simulink model "Reference_Speed_Generator"  (R2016b)
settings: Solver=FixedStepAuto  StartTime=0.0  StopTime=1500  FixedStep=0.001  RelTol=1e-3
PostLoadFcn:
  | addpath('./GUIFiles');
  | 
  | load default_gui_data.mat
  | 
  | %Load GUI
  | h_sync_gui = optiTruckGUI;
InitFcn:
  | % Call parameters initialization function
  | % run optiTruck_init_sim.m;
StopFcn:
  | %optiTruck_post_sim;
  | %optiTruck_plot_sim;
undefined symbols (not defined in the file or in its folder): DiscIntNeverNeededParam
settings Model: Creator=engin  LastModifiedBy=engin.ozatay
settings DataIOCC: SaveFormat=StructureWithTime  SaveOutput=off  SaveTime=off
settings OptimizationCC: BlockReduction=off  BufferReuse=off  LifeSpan=inf
settings DebuggingCC: AlgebraicLoopMsg=none  UnconnectedInputMsg=none  UnconnectedOutputMsg=none  UnconnectedLineMsg=none  SFExecutionAtInitializationDiag=none
settings HardwareCC: ProdBitPerSizeT=32  ProdBitPerPtrDiffT=32  ProdWordSize=32  ProdHWDeviceType=Specified

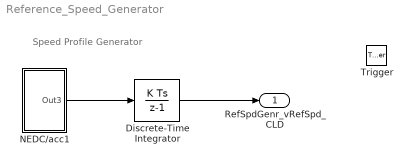
== system Reference_Speed_Generator ==
  note: Speed Profile Generator
  Trigger : TriggerPort  TriggerType=function-call  VariantControl=Variant  PortDimensions=1
  Discrete-Time Integrator : DiscreteIntegrator  SampleTime=-1  ICPrevOutput=DiscIntNeverNeededParam  ICPrevScaledInput=DiscIntNeverNeededParam
  NEDC/acc1 : Subsystem
  RefSpdGenr_vRefSpd_CLD : Outport
  wires:
  Discrete-Time Integrator/1 -> RefSpdGenr_vRefSpd_CLD/1
  NEDC/acc1/1(Out3) -> Discrete-Time Integrator/1

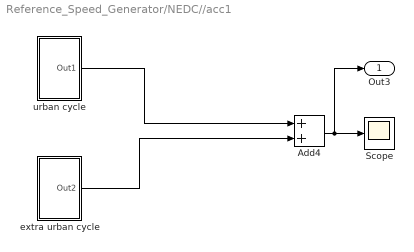
== system Reference_Speed_Generator/NEDC//acc1 ==
  Add4 : Sum
  Scope : Scope
  extra urban cycle : Subsystem
  urban cycle : Subsystem
  Out3 : Outport
  wires:
  urban cycle/1(Out1) -> Add4/1
  extra urban cycle/1(Out2) -> Add4/2
  Add4/1 -> Scope/1, Out3/1

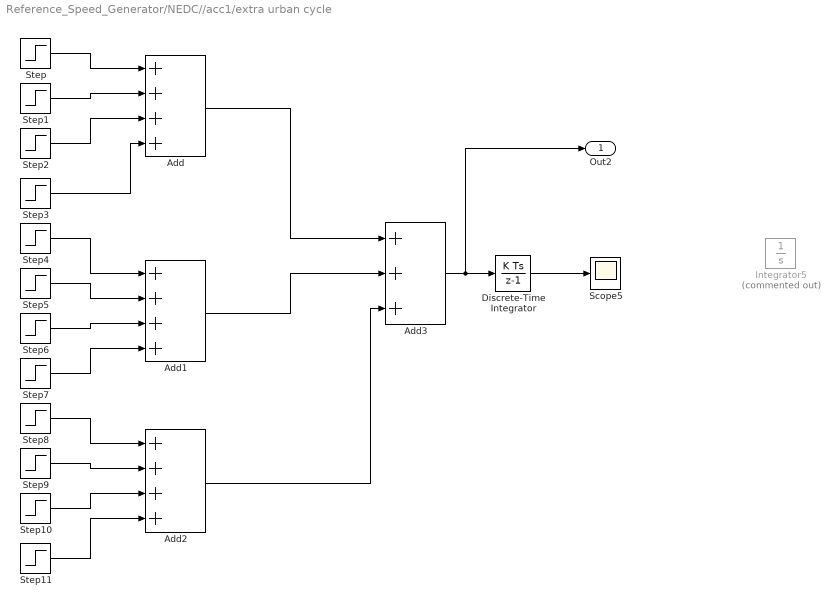
== system Reference_Speed_Generator/NEDC//acc1/extra urban cycle ==
  Add : Sum  Inputs=++++
  Add1 : Sum  Inputs=++++
  Add2 : Sum  Inputs=++++
  Add3 : Sum  Inputs=+++
  Discrete-Time Integrator : DiscreteIntegrator  SampleTime=-1  ICPrevOutput=DiscIntNeverNeededParam  ICPrevScaledInput=DiscIntNeverNeededParam
  Integrator5 : Integrator  Commented=on
  Scope5 : Scope
  Step : Step  Time=800  After=1.522/3.6  ZeroCross=off
  Step1 : Step  Time=846  After=-1.522/3.6  ZeroCross=off
  Step10 : Step  Time=1155  After=2.666/3.6  ZeroCross=off
  Step11 : Step  Time=900  After=2.5/3.6  ZeroCross=off
  Step2 : Step  Time=892  After=-2.5/3.6  ZeroCross=off
  Step3 : Step  Time=975  After=1.33/3.6  ZeroCross=off
  Step4 : Step  Time=990  After=-1.33/3.6  ZeroCross=off
  Step5 : Step  Time=1030  After=1/3.6  ZeroCross=off
  Step6 : Step  Time=1060  After=-1/3.6  ZeroCross=off
  Step7 : Step  Time=1090  After=2/3.6  ZeroCross=off
  Step8 : Step  Time=1100  After=-2/3.6  ZeroCross=off
  Step9 : Step  Time=1110  After=-2.666/3.6  ZeroCross=off
  Out2 : Outport
  wires:
  Step/1 -> Add/1
  Step1/1 -> Add/2
  Step2/1 -> Add/3
  Step3/1 -> Add/4
  Step4/1 -> Add1/1
  Step5/1 -> Add1/2
  Step6/1 -> Add1/3
  Step7/1 -> Add1/4
  Step8/1 -> Add2/1
  Step9/1 -> Add2/2
  Step10/1 -> Add2/3
  Add/1 -> Add3/1
  Add1/1 -> Add3/2
  Add2/1 -> Add3/3
  Discrete-Time Integrator/1 -> Scope5/1
  Add3/1 -> Discrete-Time Integrator/1, Out2/1
  Step11/1 -> Add2/4

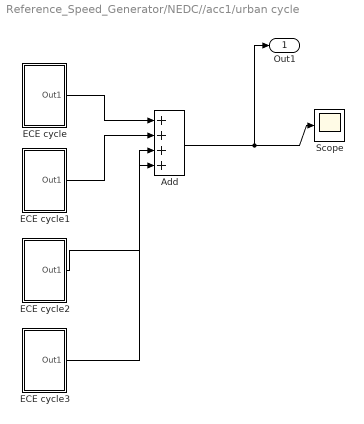
== system Reference_Speed_Generator/NEDC//acc1/urban cycle ==
  Add : Sum  Inputs=++++
  ECE cycle : Subsystem
  ECE cycle1 : Subsystem
  ECE cycle2 : Subsystem
  ECE cycle3 : Subsystem
  Scope : Scope
  Out1 : Outport
  wires:
  ECE cycle/1(Out1) -> Add/1
  ECE cycle1/1(Out1) -> Add/2
  Add/1 -> Scope/1, Out1/1
  ECE cycle2/1(Out1) -> Add/3
  ECE cycle3/1(Out1) -> Add/4

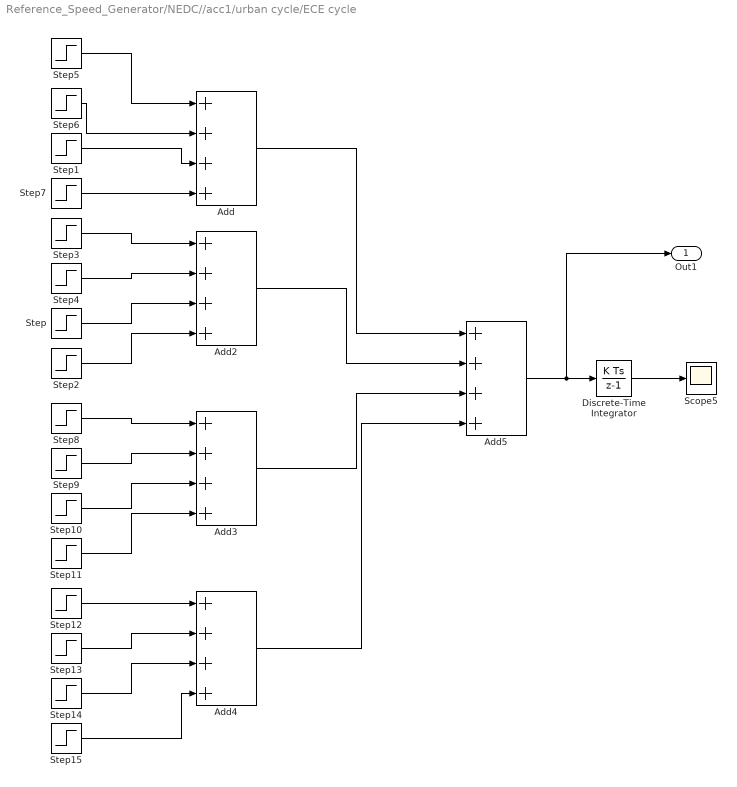
== system Reference_Speed_Generator/NEDC//acc1/urban cycle/ECE cycle ==
  Add{,2..5} (5 alike) : Sum  Inputs=++++
  Discrete-Time Integrator : DiscreteIntegrator  SampleTime=-1  ICPrevOutput=DiscIntNeverNeededParam  ICPrevScaledInput=DiscIntNeverNeededParam
  Scope5 : Scope
  Step : Step  Time=85  After=-3.2/3.6  ZeroCross=off
  Step1 : Step  Time=23  After=-3/3.6  ZeroCross=off
  Step10 : Step  Time=134  After=1.6/3.6  ZeroCross=off
  Step11 : Step  Time=144  After=-1.6/3.6  ZeroCross=off
  Step12 : Step  Time=155  After=-1.875/3.6  ZeroCross=off
  Step13 : Step  Time=163  After=1.875/3.6  ZeroCross=off
  Step14 : Step  Time=178  After=-3.5/3.6  ZeroCross=off
  Step15 : Step  Time=188  After=3.5/3.6  ZeroCross=off
  Step2 : Step  Time=95  After=3.2/3.6  ZeroCross=off
  Step3 : Step  Time=50  After=3.2/3.6  ZeroCross=off
  Step4 : Step  Time=60  After=-3.2/3.6  ZeroCross=off
  Step5 : Step  Time=10  After=3/3.6  ZeroCross=off
  Step6 : Step  Time=15  After=-3/3.6  ZeroCross=off
  Step7 : Step  Time=28  After=3/3.6  ZeroCross=off
  Step8 : Step  Time=117  After=2/3.6  ZeroCross=off
  Step9 : Step  Time=134  After=-2/3.6  ZeroCross=off
  Out1 : Outport
  wires:
  Step5/1 -> Add/1
  Step6/1 -> Add/2
  Step1/1 -> Add/3
  Step7/1 -> Add/4
  Step3/1 -> Add2/1
  Step4/1 -> Add2/2
  Step/1 -> Add2/3
  Step2/1 -> Add2/4
  Step8/1 -> Add3/1
  Step9/1 -> Add3/2
  Step10/1 -> Add3/3
  Step11/1 -> Add3/4
  Step12/1 -> Add4/1
  Step13/1 -> Add4/2
  Step14/1 -> Add4/3
  Step15/1 -> Add4/4
  Discrete-Time Integrator/1 -> Scope5/1
  Add5/1 -> Discrete-Time Integrator/1, Out1/1
  Add/1 -> Add5/1
  Add2/1 -> Add5/2
  Add3/1 -> Add5/3
  Add4/1 -> Add5/4

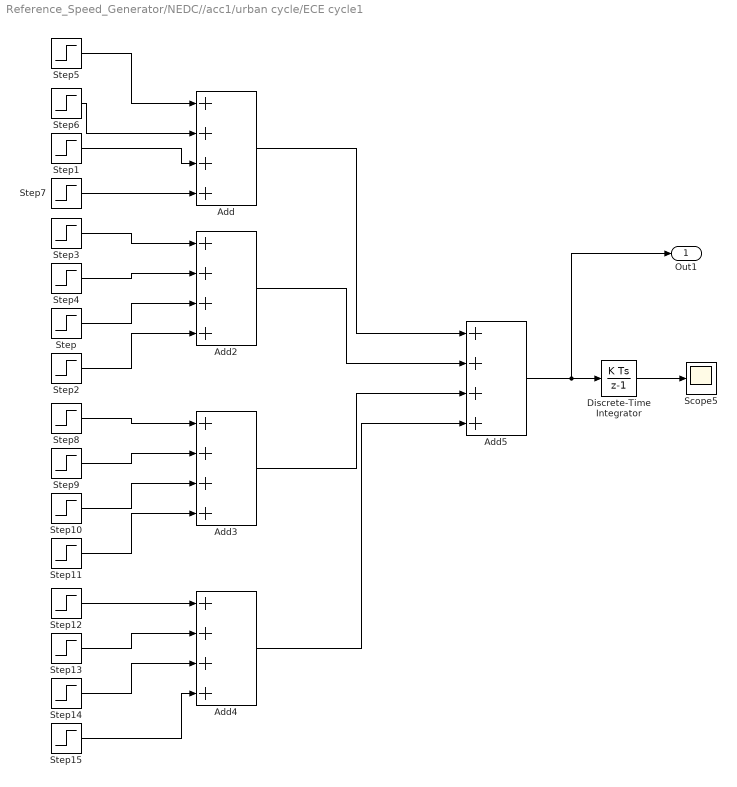
== system Reference_Speed_Generator/NEDC//acc1/urban cycle/ECE cycle1 ==
  Add{,2..5} (5 alike) : Sum  Inputs=++++
  Discrete-Time Integrator : DiscreteIntegrator  SampleTime=-1  ICPrevOutput=DiscIntNeverNeededParam  ICPrevScaledInput=DiscIntNeverNeededParam
  Scope5 : Scope
  Step : Step  Time=85+200  After=-3.2/3.6  ZeroCross=off
  Step1 : Step  Time=23+200  After=-3/3.6  ZeroCross=off
  Step10 : Step  Time=134+200  After=1.6/3.6  ZeroCross=off
  Step11 : Step  Time=144+200  After=-1.6/3.6  ZeroCross=off
  Step12 : Step  Time=155+200  After=-1.875/3.6  ZeroCross=off
  Step13 : Step  Time=163+200  After=1.875/3.6  ZeroCross=off
  Step14 : Step  Time=178+200  After=-3.5/3.6  ZeroCross=off
  Step15 : Step  Time=188+200  After=3.5/3.6  ZeroCross=off
  Step2 : Step  Time=95+200  After=3.2/3.6  ZeroCross=off
  Step3 : Step  Time=50+200  After=3.2/3.6  ZeroCross=off
  Step4 : Step  Time=60+200  After=-3.2/3.6  ZeroCross=off
  Step5 : Step  Time=10+200  After=3/3.6  ZeroCross=off
  Step6 : Step  Time=15+200  After=-3/3.6  ZeroCross=off
  Step7 : Step  Time=28+200  After=3/3.6  ZeroCross=off
  Step8 : Step  Time=117+200  After=2/3.6  ZeroCross=off
  Step9 : Step  Time=134+200  After=-2/3.6  ZeroCross=off
  Out1 : Outport
  wires:
  Step5/1 -> Add/1
  Step6/1 -> Add/2
  Step1/1 -> Add/3
  Step7/1 -> Add/4
  Step3/1 -> Add2/1
  Step4/1 -> Add2/2
  Step/1 -> Add2/3
  Step2/1 -> Add2/4
  Step8/1 -> Add3/1
  Step9/1 -> Add3/2
  Step10/1 -> Add3/3
  Step11/1 -> Add3/4
  Step12/1 -> Add4/1
  Step13/1 -> Add4/2
  Step14/1 -> Add4/3
  Step15/1 -> Add4/4
  Discrete-Time Integrator/1 -> Scope5/1
  Add5/1 -> Discrete-Time Integrator/1, Out1/1
  Add/1 -> Add5/1
  Add2/1 -> Add5/2
  Add3/1 -> Add5/3
  Add4/1 -> Add5/4

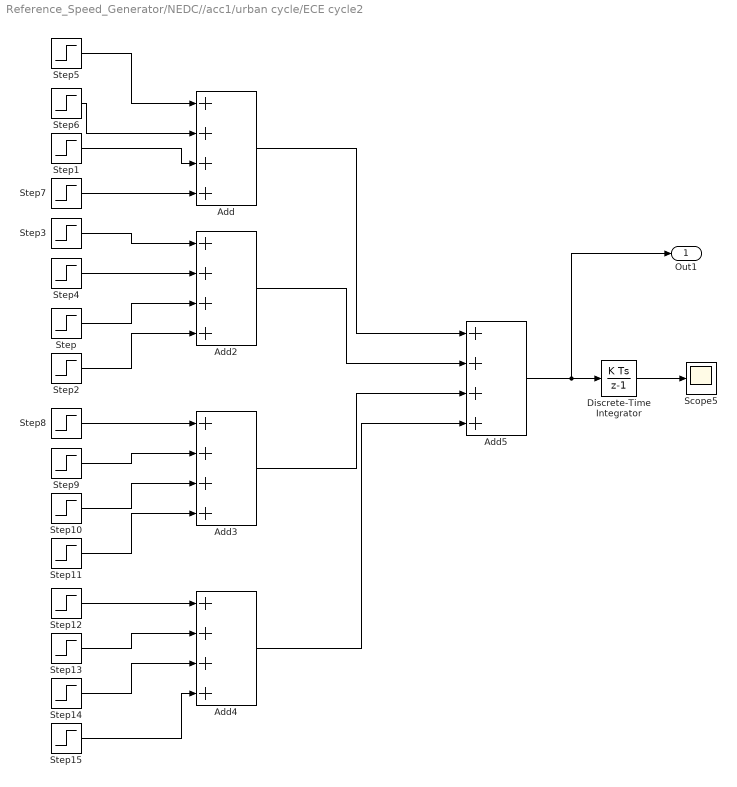
== system Reference_Speed_Generator/NEDC//acc1/urban cycle/ECE cycle2 ==
  Add{,2..5} (5 alike) : Sum  Inputs=++++
  Discrete-Time Integrator : DiscreteIntegrator  SampleTime=-1  ICPrevOutput=DiscIntNeverNeededParam  ICPrevScaledInput=DiscIntNeverNeededParam
  Scope5 : Scope
  Step : Step  Time=85+400  After=-3.2/3.6  ZeroCross=off
  Step1 : Step  Time=23+400  After=-3/3.6  ZeroCross=off
  Step10 : Step  Time=134+400  After=1.6/3.6  ZeroCross=off
  Step11 : Step  Time=144+400  After=-1.6/3.6  ZeroCross=off
  Step12 : Step  Time=155+400  After=-1.875/3.6  ZeroCross=off
  Step13 : Step  Time=163+400  After=1.875/3.6  ZeroCross=off
  Step14 : Step  Time=178+400  After=-3.5/3.6  ZeroCross=off
  Step15 : Step  Time=188+400  After=3.5/3.6  ZeroCross=off
  Step2 : Step  Time=95+400  After=3.2/3.6  ZeroCross=off
  Step3 : Step  Time=50+400  After=3.2/3.6  ZeroCross=off
  Step4 : Step  Time=60+400  After=-3.2/3.6  ZeroCross=off
  Step5 : Step  Time=10+400  After=3/3.6  ZeroCross=off
  Step6 : Step  Time=15+400  After=-3/3.6  ZeroCross=off
  Step7 : Step  Time=28+400  After=3/3.6  ZeroCross=off
  Step8 : Step  Time=117+400  After=2/3.6  ZeroCross=off
  Step9 : Step  Time=134+400  After=-2/3.6  ZeroCross=off
  Out1 : Outport
  wires:
  Step5/1 -> Add/1
  Step6/1 -> Add/2
  Step1/1 -> Add/3
  Step7/1 -> Add/4
  Step3/1 -> Add2/1
  Step4/1 -> Add2/2
  Step/1 -> Add2/3
  Step2/1 -> Add2/4
  Step8/1 -> Add3/1
  Step9/1 -> Add3/2
  Step10/1 -> Add3/3
  Step11/1 -> Add3/4
  Step12/1 -> Add4/1
  Step13/1 -> Add4/2
  Step14/1 -> Add4/3
  Step15/1 -> Add4/4
  Discrete-Time Integrator/1 -> Scope5/1
  Add5/1 -> Discrete-Time Integrator/1, Out1/1
  Add/1 -> Add5/1
  Add2/1 -> Add5/2
  Add3/1 -> Add5/3
  Add4/1 -> Add5/4

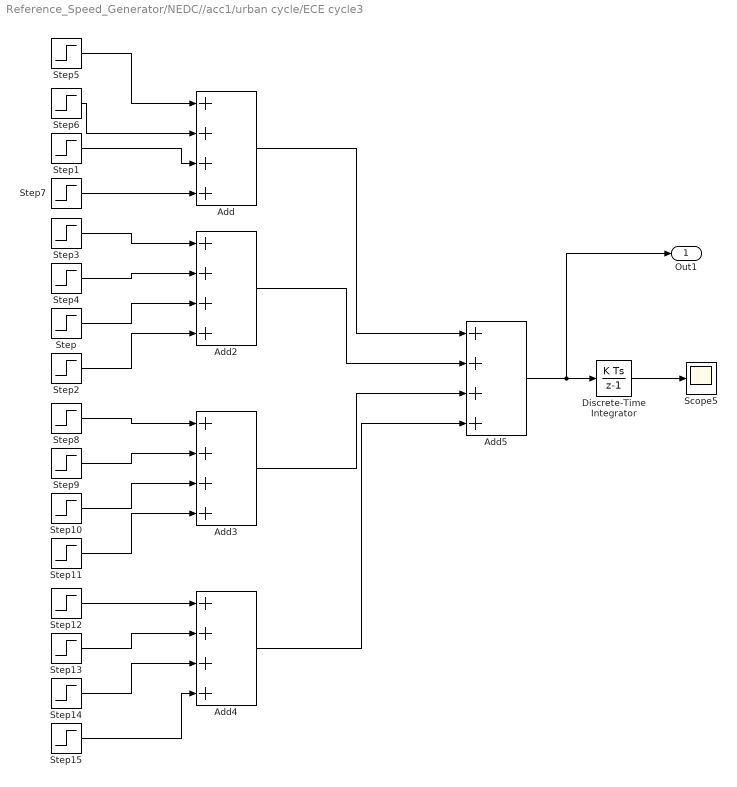
== system Reference_Speed_Generator/NEDC//acc1/urban cycle/ECE cycle3 ==
  Add{,2..5} (5 alike) : Sum  Inputs=++++
  Discrete-Time Integrator : DiscreteIntegrator  SampleTime=-1  ICPrevOutput=DiscIntNeverNeededParam  ICPrevScaledInput=DiscIntNeverNeededParam
  Scope5 : Scope
  Step : Step  Time=85+600  After=-3.2/3.6  ZeroCross=off
  Step1 : Step  Time=23+600  After=-3/3.6  ZeroCross=off
  Step10 : Step  Time=134+600  After=1.6/3.6  ZeroCross=off
  Step11 : Step  Time=144+600  After=-1.6/3.6
  Step12 : Step  Time=155+600  After=-1.875/3.6  ZeroCross=off
  Step13 : Step  Time=163+600  After=1.875/3.6  ZeroCross=off
  Step14 : Step  Time=178+600  After=-3.5/3.6  ZeroCross=off
  Step15 : Step  Time=188+600  After=3.5/3.6  ZeroCross=off
  Step2 : Step  Time=95+600  After=3.2/3.6  ZeroCross=off
  Step3 : Step  Time=50+600  After=3.2/3.6  ZeroCross=off
  Step4 : Step  Time=60+600  After=-3.2/3.6  ZeroCross=off
  Step5 : Step  Time=10+600  After=3/3.6  ZeroCross=off
  Step6 : Step  Time=15+600  After=-3/3.6  ZeroCross=off
  Step7 : Step  Time=28+600  After=3/3.6  ZeroCross=off
  Step8 : Step  Time=117+600  After=2/3.6  ZeroCross=off
  Step9 : Step  Time=134+600  After=-2/3.6  ZeroCross=off
  Out1 : Outport
  wires:
  Step5/1 -> Add/1
  Step6/1 -> Add/2
  Step1/1 -> Add/3
  Step7/1 -> Add/4
  Step3/1 -> Add2/1
  Step4/1 -> Add2/2
  Step/1 -> Add2/3
  Step2/1 -> Add2/4
  Step8/1 -> Add3/1
  Step9/1 -> Add3/2
  Step10/1 -> Add3/3
  Step11/1 -> Add3/4
  Step12/1 -> Add4/1
  Step13/1 -> Add4/2
  Step14/1 -> Add4/3
  Step15/1 -> Add4/4
  Discrete-Time Integrator/1 -> Scope5/1
  Add5/1 -> Discrete-Time Integrator/1, Out1/1
  Add/1 -> Add5/1
  Add2/1 -> Add5/2
  Add3/1 -> Add5/3
  Add4/1 -> Add5/4
